simulink model "double_pend"  (R2021a)
settings: Solver=FixedStepAuto  StartTime=0.0  StopTime=10  FixedStep=.01  RelTol=1e-3
values from neighbouring files (symbols this model uses):
  alpha = params.test_25(7,1).Value    [no_exo.m]    (also in non_same_length.m = [15,15]; play_file.m = params.test_22(7,1).Value; play_file22.m = params.test_22(7,1).Value; play_file23.m = params.test_23(7,1).Value)
  beta = params.test_25(5,1).Value    [no_exo.m]    (also in non_same_length.m = [ 1/8 ; 1/8]; play_file.m = params.test_22(5,1).Value; play_file22.m = params.test_22(5,1).Value; play_file23.m = params.test_23(5,1).Value)
  Bn0 = params.test_25(1,1).Value    [no_exo.m]    (also in non_same_length.m = [500  500]; play_file.m = params.test_22(1,1).Value; play_file22.m = params.test_22(1,1).Value; play_file23.m = params.test_23(1,1).Value)
  Bp0 = params.test_25(2,1).Value    [no_exo.m]    (also in non_same_length.m = [500  500]; play_file.m = params.test_22(2,1).Value; play_file22.m = params.test_22(2,1).Value; play_file23.m = params.test_23(2,1).Value)
  dampener = [100, 0; 0, 100]    [no_exo.m]    (also in non_same_length.m; play_file.m; play_file22.m; play_file23.m)
  Dm1 = [1000,0;0,103.228187679703]    [no_exo.m]    (also in non_same_length.m = [30,0;0,30]; play_file.m = [30,0;0,30]; play_file22.m = [300,0;0,300]; play_file23.m = [30,0;0,30])
  exo_sat = 0.0    (= 0)    [no_exo.m]    (also in non_same_length.m = 150; play_file.m = 150; play_file22.m = 150; play_file23.m = 150)
  gamma = params.test_25(9,1).Value    [no_exo.m]    (also in non_same_length.m = [15,15]; play_file.m = params.test_22(9,1).Value; play_file22.m = params.test_22(9,1).Value; play_file23.m = params.test_23(9,1).Value)
  human_sat = 150    [no_exo.m]    (also in non_same_length.m = 30; play_file.m = 30; play_file22.m = 30; play_file23.m = 200)
  Ked = [ 50, 0; 0, 50]    [no_exo.m]    (also in non_same_length.m; play_file.m; play_file22.m; play_file23.m)
  Kem = [ 50, 0; 0, 50]    [no_exo.m]    (also in non_same_length.m; play_file.m; play_file22.m; play_file23.m)
  Km1 = [1000,0;0,1000]    [no_exo.m]    (also in non_same_length.m = [30, 0; 0 30]; play_file.m = [30, 0; 0 30]; play_file22.m = [300, 0; 0 300]; play_file23.m = [30, 0; 0 30])
  Kn0 = params.test_25(3,1).Value    [no_exo.m]    (also in non_same_length.m = [500  500]; play_file.m = params.test_22(3,1).Value; play_file22.m = params.test_22(3,1).Value; play_file23.m = params.test_23(3,1).Value)
  Kp0 = params.test_25(4,1).Value    [no_exo.m]    (also in non_same_length.m = [500 500]; play_file.m = params.test_22(4,1).Value; play_file22.m = params.test_22(4,1).Value; play_file23.m = params.test_23(4,1).Value)
  l = [0.324, 0.3900]    [myStateTransitionFcn.m]
  lambda2 = params.test_25(6,1).Value    [no_exo.m]    (also in non_same_length.m = [1.2, 0; 0 1.25]; play_file.m = params.test_22(6,1).Value; play_file22.m = params.test_22(6,1).Value; play_file23.m = params.test_23(6,1).Value)
  le = [0.324, 0.3900]    [no_exo.m]    (also in non_same_length.m; play_file.m; play_file22.m; play_file23.m)
  lh = [0.324, 0.3900]    [no_exo.m]    (also in non_same_length.m; play_file.m; play_file22.m; play_file23.m)
  Md = [10.0, 0; 0, 10.0]    [no_exo.m]    (also in non_same_length.m; play_file.m; play_file22.m; play_file23.m)
  me = [ 2.11, 1.28]  + mh    [no_exo.m]    (also in non_same_length.m; play_file.m; play_file22.m; play_file23.m)
  mh = [11.824, 3.848]    [no_exo.m]    (also in non_same_length.m; play_file.m; play_file22.m; play_file23.m)
  rho2 = params.test_25(8,1).Value    [no_exo.m]    (also in non_same_length.m = [100, 0; 0, 450]; play_file.m = params.test_22(8,1).Value; play_file22.m = params.test_22(8,1).Value; play_file23.m = params.test_23(8,1).Value)
  spring = [100, 0; 0, 100]    [no_exo.m]    (also in non_same_length.m; play_file.m; play_file22.m; play_file23.m)
undefined symbols (not defined in the file or in its folder): l1, l2, me2
libraries: sharedTrackingLibrary x2, simulink x2, robotcorelib x1
settings Model: Creator=nathanielgoldfarb  LastModifiedBy=nathanielgoldfarb
settings SolverCC: AlgebraicLoopSolver=TrustRegion
settings DataIOCC: ReturnWorkspaceOutputsName=SDOSimTest_Log
settings DebuggingCC: SFMachineParentedDataDiag=warning

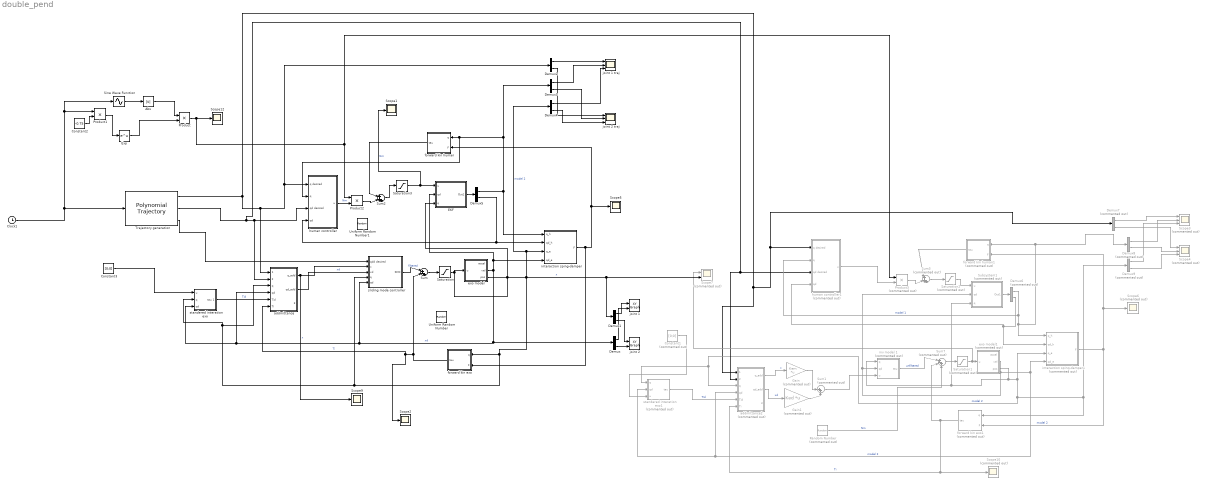
== system double_pend ==
  " interaction sping-damper" : Subsystem
  " interaction sping-damper1" : Subsystem  Commented=on
  Abs : Abs
  Clock1 : Clock
  Constant1 : Constant  Commented=on  Value=[0;0]
  Constant2 : Constant  Value=-0.75
  Constant3 : Constant  Value=[0;0]
  Demux{,1..5} (6 alike) : Demux  Outputs=2
  Demux{6..9} (4 alike) : Demux  Commented=on  Outputs=2
  EKF : Subsystem
  Exp : Math  SaturateOnIntegerOverflow=on
  Gain : Gain  Commented=on  Gain=Kem  Multiplication=Matrix(K*u)
  Gain1 : Gain  Commented=on  Gain=Ked  Multiplication=Matrix(K*u)
  Product : Product
  Product1 : Product
  Product2 : Product
  Product3 : Product  Commented=on
  Random Number : RandomNumber  Commented=on  Variance=15  SampleTime=0.1
  Saturation : Saturate  UpperLimit=exo_sat  LowerLimit=-exo_sat
  Saturation1 : Saturate  Commented=on  UpperLimit=exo_sat  LowerLimit=-exo_sat
  Saturation2 : Saturate  Commented=on  UpperLimit=human_sat  LowerLimit=-human_sat
  Saturation3 : Saturate  UpperLimit=human_sat  LowerLimit=-human_sat
  Scope{1..2,5,9,12} (5 alike) : Scope
  Scope10 : Scope  Commented=on
  Scope3 : Scope  Commented=on  NumInputPorts=3
  Scope4 : Scope  Commented=on  NumInputPorts=3
  Scope6 : Scope  Commented=on
  Scope7 : Scope  Commented=on  NumInputPorts=2
  Sine Wave Function : Sin  TimeSource=Use external signal  Frequency=5  SampleTime=0
  Subsystem1 : Subsystem  Commented=on
  Sum : Sum  Inputs=|+-+
  Sum1 : Sum  Commented=on  Inputs=|++
  Sum2 : Sum  Inputs=|+++
  Sum3 : Sum  Commented=on  Inputs=|+++
  Sum7 : Sum  Commented=on  Inputs=|+-+
  Trajectory generation : robotcorelib/Polynomial Trajectory  WaypointSource=Internal  Waypoints="[ 0 , -pi, 0;  0 -0.5*pi,0 ]"  TimePoints=[ 0, 5, 10]  TimeInterval=[ 1, 4 ]  Method=Cubic Polynomial  ParameterSource=Internal  VelocityBoundaryCondition=zeros( 2, 3 )  AccelerationBoundaryCondition=zeros( 2, 5 )  SimulateUsing=Interpreted execution
  Uniform Random Number : UniformRandomNumber  Minimum=-5  Maximum=5  SampleTime=0.1
  Uniform Random Number1 : UniformRandomNumber  Minimum=-5  Maximum=5  SampleTime=0.1
  addmittance : Subsystem
  addmittance2 : Subsystem  Commented=on
  exo model : Subsystem
  exo model1 : Subsystem  Commented=on
  forward kin exo : Subsystem
  forward kin exo1 : Subsystem  Commented=on
  forward kin human : Subsystem
  forward kin human1 : Subsystem  Commented=on
  human controller : Subsystem
  human controller1 : Subsystem  Commented=on
  inv model 1 : Subsystem  Commented=on
  joint 1 : simulink/Sinks/XY Graph  xmin=-15  xmax=15  ymin=-10  ymax=10  st=-1
  joint 1 traj : Scope  NumInputPorts=3
  joint 2 : simulink/Sinks/XY Graph  xmin=-10  xmax=10  ymin=-10  ymax=10  st=-1
  joint 2 traj : Scope  NumInputPorts=3
  sliding mode controller : Subsystem
  standered interation exo : Subsystem
  standered interation exo1 : Subsystem  Commented=on
  wires:
  forward kin human/1(tau) -> Sum2/1
  Demux4/2 -> joint 2 traj/3
  addmittance/2(qd_add) -> sliding mode controller/3(xd)  "xd"
  Constant1/1 -> standered interation exo1/3("u ")
  Demux9/2 -> Scope4/3
  Trajectory generation/3 -> sliding mode controller/1(qdd desired)
  addmittance2/1(q_add) -> Gain/1  "x"
  inv model 1/1("tau ") -> Sum7/1  "unfiltered"
  Demux3/1 -> joint 1 traj/2
  Clock1/1 -> Trajectory generation/1, Sine Wave Function/1, Product1/1
  Demux7/2 -> Scope4/1
  " interaction sping-damper"/1(F) -> forward kin exo/2(F), forward kin human/2(F), Scope5/1
  Demux2/1 -> joint 1 traj/1
  Gain/1 -> Sum1/1
  " interaction sping-damper1"/1(F) -> forward kin exo1/2(F), forward kin human1/2(F), Scope6/1  "model 2"
  exo model1/2(vel) -> inv model 1/2(qd), Subsystem1/2(qd), " interaction sping-damper1"/4("qd_e "), addmittance2/4(qd), standered interation exo1/2(qd)  "model 2"
  Gain1/1 -> Sum1/2
  Sum1/1 -> inv model 1/3("u ")
  Demux9/1 -> Scope3/3
  forward kin human1/1(tau) -> Sum3/1
  Sum7/1 -> Saturation1/1
  Demux4/1 -> joint 1 traj/3
  standered interation exo/1(tau 1) -> addmittance/5(Tid)  "Tid"
  Demux8/1 -> Scope3/2
  addmittance2/2(qd_add) -> Gain1/1  "xd"
  Random Number/1 -> Sum7/3  "Nm"
  Trajectory generation/1 -> addmittance/1(q desird), human controller/1(q desired), Demux2/1, addmittance2/1(q desird), human controller1/1(q desired), Demux7/1
  sliding mode controller/1(SMC) -> Sum/1  "filtered"
  exo model1/3(pos) -> Subsystem1/3(q), inv model 1/1(q), " interaction sping-damper1"/3(q_e), addmittance2/3(q), standered interation exo1/1(q), Demux9/1, forward kin exo1/1(q)  "model 2"
  Demux3/2 -> joint 2 traj/2
  Demux7/1 -> Scope3/1
  Demux6/2 -> human controller1/4(qd), " interaction sping-damper1"/2(qd_h)
  standered interation exo1/1("tau ") -> addmittance2/5(Tid)  "Tid"
  forward kin exo/1(tau) -> addmittance/6(Ti), Scope2/1, Sum/2  "Ti"
  Sum3/1 -> Saturation2/1
  Trajectory generation/2 -> addmittance2/2(qd desird), human controller1/3(qd desired), human controller/3(qd desired), addmittance/2(qd desird)
  addmittance/1(q_add) -> Scope9/1, sliding mode controller/2(x)  "x"
  Demux8/2 -> Scope4/2
  Demux6/1 -> " interaction sping-damper1"/1(q_h), forward kin human1/1(q), Demux8/1, human controller1/2(q)  "model 1"
  exo model/3(pos) -> Demux4/1, " interaction sping-damper"/3(q_e), sliding mode controller/4(q), standered interation exo/2(q), addmittance/3(q), forward kin exo/1(q), EKF/3(q)  "model 2"
  Demux2/2 -> joint 2 traj/1
  Demux5/1 -> Demux3/1, human controller/2(q), forward kin human/1(q), " interaction sping-damper"/1(q_h)
  Demux5/2 -> human controller/4(qd), " interaction sping-damper"/2(qd_h)
  Sum2/1 -> Saturation3/1
  EKF/1(Out1) -> Demux5/1
  Subsystem1/1(Out1) -> Demux6/1
  Sum/1 -> Saturation/1
  Saturation1/1 -> Scope7/1, exo model1/1(u)
  Saturation2/1 -> Subsystem1/1(u)
  Saturation3/1 -> Scope1/1, EKF/1(u)  "Nm"
  Abs/1 -> Product/1
  Sine Wave Function/1 -> Abs/1
  Product1/1 -> Exp/1
  Constant2/1 -> Product1/2
  Exp/1 -> Product/2
  human controller/1(u) -> Product2/2  "Nm"
  Product2/1 -> Sum2/2
  human controller1/1(u) -> Product3/2
  Product3/1 -> Sum3/2
  Product/1 -> Product2/1, Product3/1, Scope12/1
  forward kin exo1/1(tau) -> Sum7/2, addmittance2/6(Ti), Scope10/1  "Ti"
  Constant3/1 -> standered interation exo/1(u)
  Demux/2 -> joint 2/2
  Saturation/1 -> Demux1/1, Scope7/2, exo model/1(u)  "x"
  Demux1/2 -> joint 2/1
  Demux1/1 -> joint 1/1
  exo model/2(vel) -> Demux/1, addmittance/4(qd), standered interation exo/3(qd), sliding mode controller/5(qd), EKF/2(qd), " interaction sping-damper"/4("qd_e ")  "xd"
  Demux/1 -> joint 1/2

== system double_pend/ interaction sping-damper ==
  q_h : Inport
  qd_h : Inport  Port=2
  q_e : Inport  Port=3
  "qd_e " : Inport  Port=4
  Mux : Mux  Inputs=2
  Subsystem : Subsystem
  Subsystem1 : Subsystem
  forward kin : Subsystem
  forward kin1 : Subsystem
  F : Outport
  wires:
  qd_h/1 -> forward kin/2(qd)
  q_h/1 -> forward kin/1("q ")
  "qd_e "/1 -> forward kin1/2(qd)
  q_e/1 -> forward kin1/1("q ")
  forward kin/1(pos1) -> Subsystem/1(x human)
  forward kin/3(vel1) -> Subsystem/2("xd human ")
  forward kin1/1(pos1) -> Subsystem/3(x exo)
  forward kin1/3(vel1) -> Subsystem/4(xd exo)
  forward kin/2(pos2) -> Subsystem1/1(x human)
  forward kin1/2(pos2) -> Subsystem1/3(x exo)
  forward kin/4(vel2) -> Subsystem1/2("xd human ")
  forward kin1/4(vel2) -> Subsystem1/4(xd exo)
  Subsystem/1(F) -> Mux/1
  Subsystem1/1(F) -> Mux/2
  Mux/1 -> F/1

== system double_pend/ interaction sping-damper1 ==
  q_h : Inport
  qd_h : Inport  Port=2
  q_e : Inport  Port=3
  "qd_e " : Inport  Port=4
  Mux : Mux  Inputs=2
  Subsystem : Subsystem
  Subsystem1 : Subsystem
  forward kin : Subsystem
  forward kin2 : Subsystem
  F : Outport
  wires:
  qd_h/1 -> forward kin/2(qd)
  q_h/1 -> forward kin/1("q ")
  "qd_e "/1 -> forward kin2/2(qd)
  q_e/1 -> forward kin2/1("q ")
  forward kin/1(pos1) -> Subsystem/1(x human)
  forward kin/3(vel1) -> Subsystem/2("xd human ")
  forward kin2/1(pos1) -> Subsystem/3(x exo)
  forward kin2/3(vel1) -> Subsystem/4(xd exo)
  forward kin/2(pos2) -> Subsystem1/1(x human)
  forward kin2/2(pos2) -> Subsystem1/3(x exo)
  forward kin/4(vel2) -> Subsystem1/2("xd human ")
  forward kin2/4(vel2) -> Subsystem1/4(xd exo)
  Subsystem/1(F) -> Mux/1
  Subsystem1/1(F) -> Mux/2
  Mux/1 -> F/1

== system double_pend/EKF ==
  u : Inport
  qd : Inport  Port=2
  q : Inport  Port=3
  Constant5 : Constant
  Extended Kalman Filter : sharedTrackingLibrary/Extended Kalman Filter  StateTransitionFcn=myStateTransitionFcn  HasStateTransitionJacobianFcn=off  HasAdditiveProcessNoise=Additive  ProcessNoise=myQ  HasTimeVaryingProcessNoise=off  HasStateTransitionFcnExtraArgument=1  InitialState=[0;0;0;0]  InitialStateCovariance=1  MeasurementFcn1=myMeasurementFcn  HasMeasurementJacobianFcn1=off  HasMeasurementEnablePort1=on  HasAdditiveMeasurementNoise1=Additive  MeasurementNoise1=myR  HasTimeVaryingMeasurementNoise1=off  HasMeasurementFcnExtraArgument1=0  MeasurementFcn2=myMeasurementFcn  HasMeasurementJacobianFcn2=off  HasMeasurementEnablePort2=off  HasAdditiveMeasurementNoise2=Additive  MeasurementNoise2=1  HasTimeVaryingMeasurementNoise2=off  HasMeasurementFcnExtraArgument2=0  MeasurementFcn3=myMeasurementFcn  HasMeasurementJacobianFcn3=off  HasMeasurementEnablePort3=off  HasAdditiveMeasurementNoise3=Additive  MeasurementNoise3=1  HasTimeVaryingMeasurementNoise3=off  HasMeasurementFcnExtraArgument3=0  MeasurementFcn4=myMeasurementFcn  HasMeasurementJacobianFcn4=off  HasMeasurementEnablePort4=off  HasAdditiveMeasurementNoise4=Additive  MeasurementNoise4=1  HasTimeVaryingMeasurementNoise4=off  HasMeasurementFcnExtraArgument4=0  MeasurementFcn5=myMeasurementFcn  HasMeasurementJacobianFcn5=off  HasMeasurementEnablePort5=off  HasAdditiveMeasurementNoise5=Additive  MeasurementNoise5=1  HasTimeVaryingMeasurementNoise5=off  HasMeasurementFcnExtraArgument5=0  EnableMultirate=off  StateTransitionFcnSampleTime=1  MeasurementFcn1SampleTime=1  MeasurementFcn2SampleTime=1  MeasurementFcn3SampleTime=1  MeasurementFcn4SampleTime=1  MeasurementFcn5SampleTime=1  UseCurrentEstimator=on  OutputStateCovariance=off  DataType=double  SampleTime=.01  NumberOfMeasurements=1
      settings: SourceProductBaseCode=CT,DR,TF,ID,LP,NV,AR,RO,RR,UV,VE
  Mux : Mux  Inputs=2
  Zero-Order Hold : ZeroOrderHold  SampleTime=.01
  Zero-Order Hold1 : ZeroOrderHold  SampleTime=.01
  Out1 : Outport
  wires:
  Mux/1 -> Zero-Order Hold/1
  Zero-Order Hold/1 -> Extended Kalman Filter/3
  Zero-Order Hold1/1 -> Extended Kalman Filter/1
  u/1 -> Zero-Order Hold1/1
  Constant5/1 -> Extended Kalman Filter/2
  Extended Kalman Filter/1 -> Out1/1
  q/1 -> Mux/1
  qd/1 -> Mux/2

== system double_pend/Subsystem1 ==
  u : Inport
  qd : Inport  Port=2
  q : Inport  Port=3
  Constant5 : Constant
  Extended Kalman Filter : sharedTrackingLibrary/Extended Kalman Filter  StateTransitionFcn=myStateTransitionFcn  HasStateTransitionJacobianFcn=off  HasAdditiveProcessNoise=Additive  ProcessNoise=myQ  HasTimeVaryingProcessNoise=off  HasStateTransitionFcnExtraArgument=1  InitialState=[0;0;0;0]  InitialStateCovariance=1  MeasurementFcn1=myMeasurementFcn  HasMeasurementJacobianFcn1=off  HasMeasurementEnablePort1=on  HasAdditiveMeasurementNoise1=Additive  MeasurementNoise1=myR  HasTimeVaryingMeasurementNoise1=off  HasMeasurementFcnExtraArgument1=0  MeasurementFcn2=myMeasurementFcn  HasMeasurementJacobianFcn2=off  HasMeasurementEnablePort2=off  HasAdditiveMeasurementNoise2=Additive  MeasurementNoise2=1  HasTimeVaryingMeasurementNoise2=off  HasMeasurementFcnExtraArgument2=0  MeasurementFcn3=myMeasurementFcn  HasMeasurementJacobianFcn3=off  HasMeasurementEnablePort3=off  HasAdditiveMeasurementNoise3=Additive  MeasurementNoise3=1  HasTimeVaryingMeasurementNoise3=off  HasMeasurementFcnExtraArgument3=0  MeasurementFcn4=myMeasurementFcn  HasMeasurementJacobianFcn4=off  HasMeasurementEnablePort4=off  HasAdditiveMeasurementNoise4=Additive  MeasurementNoise4=1  HasTimeVaryingMeasurementNoise4=off  HasMeasurementFcnExtraArgument4=0  MeasurementFcn5=myMeasurementFcn  HasMeasurementJacobianFcn5=off  HasMeasurementEnablePort5=off  HasAdditiveMeasurementNoise5=Additive  MeasurementNoise5=1  HasTimeVaryingMeasurementNoise5=off  HasMeasurementFcnExtraArgument5=0  EnableMultirate=off  StateTransitionFcnSampleTime=1  MeasurementFcn1SampleTime=1  MeasurementFcn2SampleTime=1  MeasurementFcn3SampleTime=1  MeasurementFcn4SampleTime=1  MeasurementFcn5SampleTime=1  UseCurrentEstimator=on  OutputStateCovariance=off  DataType=double  SampleTime=.01  NumberOfMeasurements=1
      settings: SourceProductBaseCode=CT,DR,TF,ID,LP,NV,AR,RO,RR,UV,VE
  Mux : Mux  Inputs=2
  Zero-Order Hold : ZeroOrderHold  SampleTime=.01
  Zero-Order Hold1 : ZeroOrderHold  SampleTime=.01
  Out1 : Outport
  wires:
  Mux/1 -> Zero-Order Hold/1
  Zero-Order Hold/1 -> Extended Kalman Filter/3
  Zero-Order Hold1/1 -> Extended Kalman Filter/1
  u/1 -> Zero-Order Hold1/1
  Constant5/1 -> Extended Kalman Filter/2
  Extended Kalman Filter/1 -> Out1/1
  q/1 -> Mux/1
  qd/1 -> Mux/2

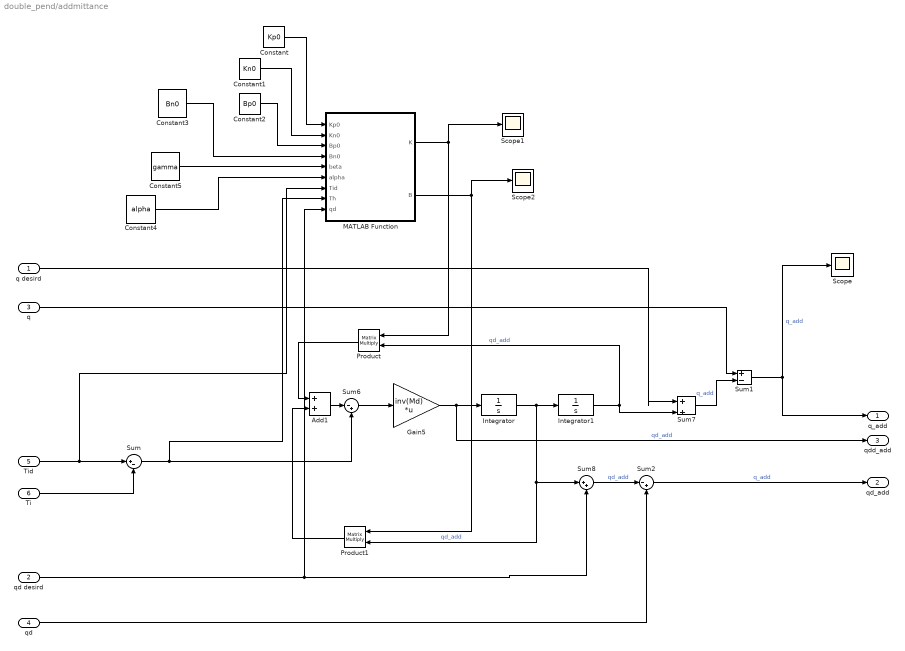
== system double_pend/addmittance ==
  q desird : Inport
  qd desird : Inport  Port=2
  q : Inport  Port=3
  qd : Inport  Port=4
  Tid : Inport  Port=5
  Ti : Inport  Port=6
  Add1 : Sum
  Constant : Constant  Value=Kp0
  Constant1 : Constant  Value=Kn0
  Constant2 : Constant  Value=Bp0
  Constant3 : Constant  Value=Bn0
  Constant4 : Constant  Value=alpha
  Constant5 : Constant  Value=gamma
  Gain5 : Gain  Gain=inv(Md)  Multiplication=Matrix(K*u)
  Integrator : Integrator
  Integrator1 : Integrator  InitialCondition=[pi;0.5*pi]
  MATLAB Function : MATLAB Function  TreatAsAtomicUnit=on
  Product : Product  Multiplication=Matrix(*)
  Product1 : Product  Multiplication=Matrix(*)
  Scope : Scope
  Scope1 : Scope
  Scope2 : Scope
  Sum : Sum  Inputs=|+-
  Sum1 : Sum  Inputs=|+-
  Sum2 : Sum  Inputs=|-+
  Sum6 : Sum  Inputs=|-+
  Sum7 : Sum  Inputs=|++
  Sum8 : Sum  Inputs=|++
  q_add : Outport
  qd_add : Outport  Port=2
  qdd_add : Outport  Port=3
  wires:
  Add1/1 -> Sum6/1
  qd desird/1 -> MATLAB Function/9(qd), Sum8/2
  Gain5/1 -> qdd_add/1, Integrator/1  "qd_add"
  Sum6/1 -> Gain5/1
  Product/1 -> Add1/1
  q desird/1 -> Sum7/1
  qd/1 -> Sum2/2
  Sum2/1 -> qd_add/1  "q_add"
  Sum7/1 -> Sum1/2  "q_add"
  q/1 -> Sum1/1
  Sum1/1 -> q_add/1, Scope/1  "q_add"
  Sum8/1 -> Sum2/1  "qd_add"
  Integrator/1 -> Product1/2, Sum8/1, Integrator1/1  "qd_add"
  Integrator1/1 -> Product/2, Sum7/2  "qd_add"
  Sum/1 -> MATLAB Function/8(Th), Sum6/2
  Tid/1 -> MATLAB Function/7(Tid), Sum/1
  Ti/1 -> Sum/2
  Product1/1 -> Add1/2
  MATLAB Function/1(K) -> Product/1, Scope1/1
  MATLAB Function/2(B) -> Product1/1, Scope2/1
  Constant/1 -> MATLAB Function/1(Kp0)
  Constant1/1 -> MATLAB Function/2(Kn0)
  Constant2/1 -> MATLAB Function/3(Bp0)
  Constant3/1 -> MATLAB Function/4(Bn0)
  Constant4/1 -> MATLAB Function/6(alpha)
  Constant5/1 -> MATLAB Function/5(beta)

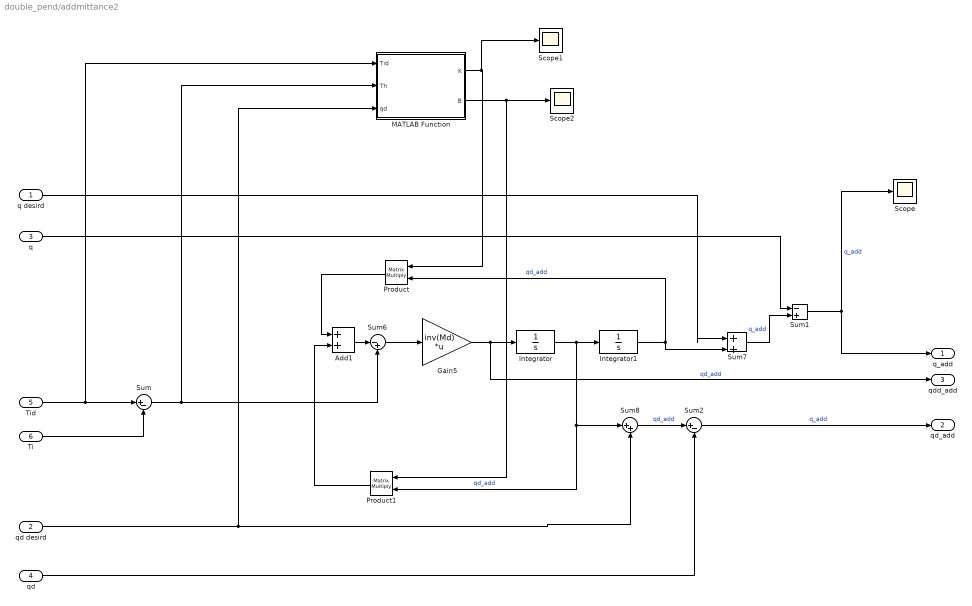
== system double_pend/addmittance2 ==
  q desird : Inport
  qd desird : Inport  Port=2
  q : Inport  Port=3
  qd : Inport  Port=4
  Tid : Inport  Port=5
  Ti : Inport  Port=6
  Add1 : Sum
  Gain5 : Gain  Gain=inv(Md)  Multiplication=Matrix(K*u)
  Integrator : Integrator
  Integrator1 : Integrator  InitialCondition=[pi;0.5*pi]
  MATLAB Function : MATLAB Function  TreatAsAtomicUnit=on
  Product : Product  Multiplication=Matrix(*)
  Product1 : Product  Multiplication=Matrix(*)
  Scope : Scope
  Scope1 : Scope
  Scope2 : Scope
  Sum : Sum  Inputs=|+-
  Sum1 : Sum  Inputs=|-+
  Sum2 : Sum  Inputs=|+-
  Sum6 : Sum  Inputs=|-+
  Sum7 : Sum  Inputs=|++
  Sum8 : Sum  Inputs=|++
  q_add : Outport
  qd_add : Outport  Port=2
  qdd_add : Outport  Port=3
  wires:
  Add1/1 -> Sum6/1
  qd desird/1 -> MATLAB Function/3(qd), Sum8/2
  Gain5/1 -> qdd_add/1, Integrator/1  "qd_add"
  Sum6/1 -> Gain5/1
  Product/1 -> Add1/1
  q desird/1 -> Sum7/1
  qd/1 -> Sum2/2
  Sum2/1 -> qd_add/1  "q_add"
  Sum7/1 -> Sum1/2  "q_add"
  q/1 -> Sum1/1
  Sum1/1 -> q_add/1, Scope/1  "q_add"
  Sum8/1 -> Sum2/1  "qd_add"
  Integrator/1 -> Product1/2, Sum8/1, Integrator1/1  "qd_add"
  Integrator1/1 -> Product/2, Sum7/2  "qd_add"
  Sum/1 -> MATLAB Function/2(Th), Sum6/2
  Tid/1 -> MATLAB Function/1(Tid), Sum/1
  Ti/1 -> Sum/2
  Product1/1 -> Add1/2
  MATLAB Function/1(K) -> Scope1/1, Product/1
  MATLAB Function/2(B) -> Scope2/1, Product1/1

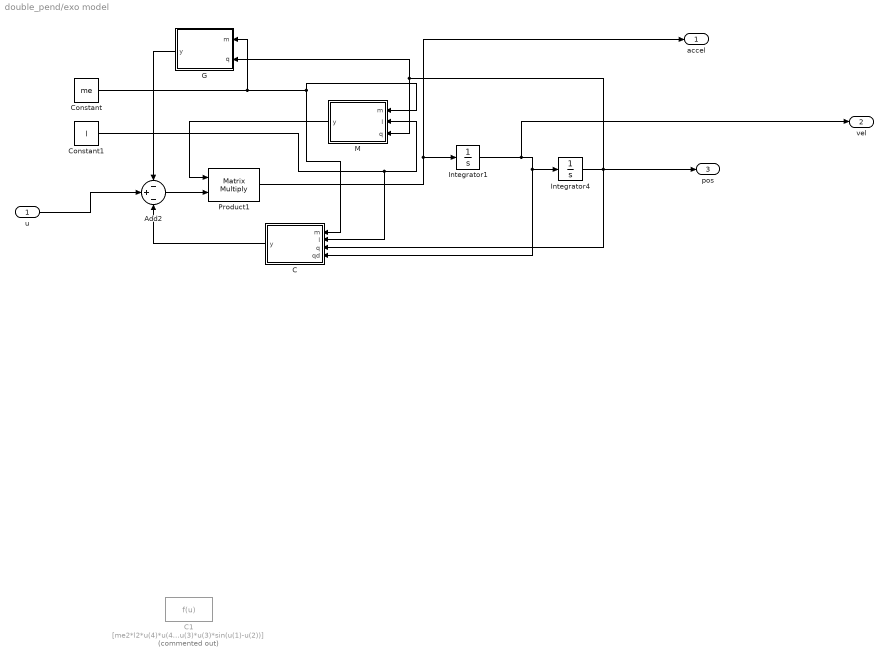
== system double_pend/exo model ==
  u : Inport
  Add2 : Sum  Inputs=-+-
  C : MATLAB Function  TreatAsAtomicUnit=on
  C1 : Fcn  Commented=on  Expr=[me2*l2*u(4)*u(4)*sin(u(1)-u(2)); -me2*l1*u(3)*u(3)*sin(u(1)-u(2))]
  Constant : Constant  Value=me
  Constant1 : Constant  Value=l
  G : MATLAB Function  TreatAsAtomicUnit=on
  Integrator1 : Integrator  InitialCondition=[0;0]
  Integrator4 : Integrator  InitialCondition=[0.01;0.01]
  M : MATLAB Function  TreatAsAtomicUnit=on
  Product1 : Product  Multiplication=Matrix(*)
  accel : Outport
  vel : Outport  Port=2
  pos : Outport  Port=3
  wires:
  Constant/1 -> G/1(m), M/1(m), C/1(m)
  M/1(y) -> Product1/1
  Add2/1 -> Product1/2
  C/1(y) -> Add2/3
  G/1(y) -> Add2/1
  u/1 -> Add2/2
  Product1/1 -> accel/1, Integrator1/1
  Constant1/1 -> C/2(l), M/2(l)
  Integrator4/1 -> C/3(q), pos/1, M/3(q), G/2(q)
  Integrator1/1 -> vel/1, C/4(qd), Integrator4/1

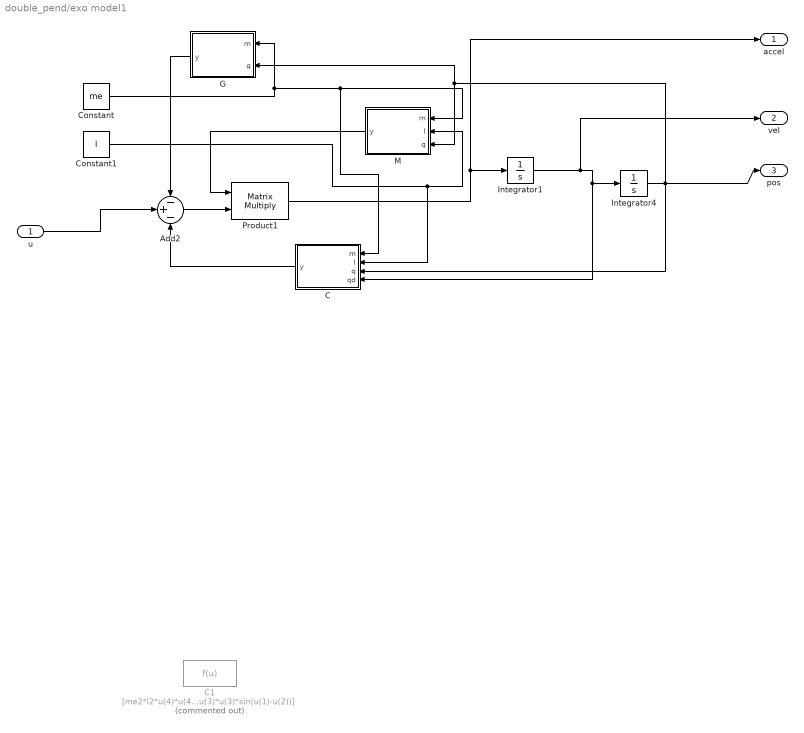
== system double_pend/exo model1 ==
  u : Inport
  Add2 : Sum  Inputs=-+-
  C : MATLAB Function  TreatAsAtomicUnit=on
  C1 : Fcn  Commented=on  Expr=[me2*l2*u(4)*u(4)*sin(u(1)-u(2)); -me2*l1*u(3)*u(3)*sin(u(1)-u(2))]
  Constant : Constant  Value=me
  Constant1 : Constant  Value=l
  G : MATLAB Function  TreatAsAtomicUnit=on
  Integrator1 : Integrator  InitialCondition=[0;0]
  Integrator4 : Integrator  InitialCondition=[0.01;0.01]
  M : MATLAB Function  TreatAsAtomicUnit=on
  Product1 : Product  Multiplication=Matrix(*)
  accel : Outport
  vel : Outport  Port=2
  pos : Outport  Port=3
  wires:
  Constant/1 -> G/1(m), C/1(m), M/1(m)
  M/1(y) -> Product1/1
  Add2/1 -> Product1/2
  C/1(y) -> Add2/3
  G/1(y) -> Add2/1
  u/1 -> Add2/2
  Product1/1 -> accel/1, Integrator1/1
  Constant1/1 -> C/2(l), M/2(l)
  Integrator1/1 -> vel/1, C/4(qd), Integrator4/1
  Integrator4/1 -> C/3(q), pos/1, M/3(q), G/2(q)

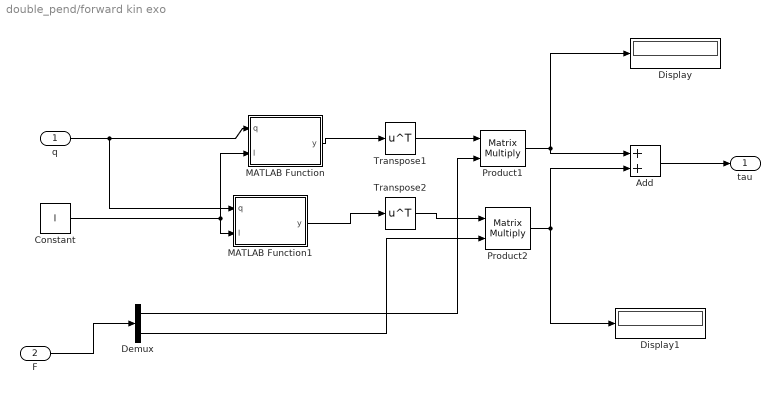
== system double_pend/forward kin exo ==
  q : Inport
  F : Inport  Port=2
  Add : Sum
  Constant : Constant  Value=l
  Demux : Demux  Outputs=2
  Display : Display
  Display1 : Display
  MATLAB Function : MATLAB Function  TreatAsAtomicUnit=on
  MATLAB Function1 : MATLAB Function  TreatAsAtomicUnit=on
  Product1 : Product  Multiplication=Matrix(*)
  Product2 : Product  Multiplication=Matrix(*)
  Transpose1 : Math  Operator=transpose  SaturateOnIntegerOverflow=on
  Transpose2 : Math  Operator=transpose  SaturateOnIntegerOverflow=on
  tau : Outport
  wires:
  Product1/1 -> Add/1, Display/1
  F/1 -> Demux/1
  q/1 -> MATLAB Function1/1(q), MATLAB Function/1(q)
  Constant/1 -> MATLAB Function/2(l), MATLAB Function1/2(l)
  Add/1 -> tau/1
  Demux/2 -> Product2/2
  Transpose2/1 -> Product2/1
  Demux/1 -> Product1/2
  Product2/1 -> Add/2, Display1/1
  MATLAB Function1/1(y) -> Transpose2/1
  MATLAB Function/1(y) -> Transpose1/1
  Transpose1/1 -> Product1/1

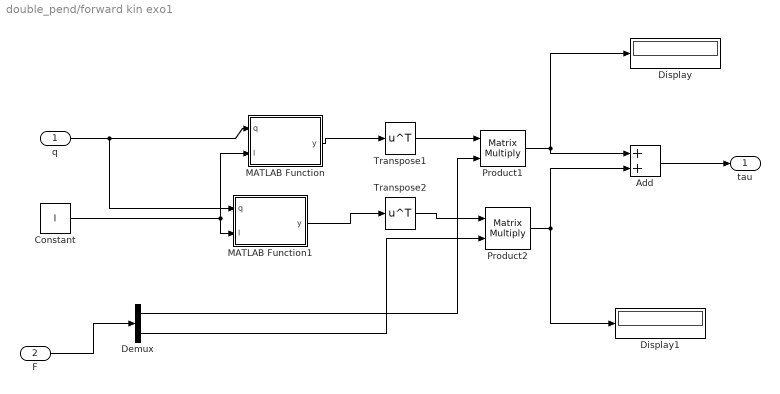
== system double_pend/forward kin exo1 ==
  q : Inport
  F : Inport  Port=2
  Add : Sum
  Constant : Constant  Value=l
  Demux : Demux  Outputs=2
  Display : Display
  Display1 : Display
  MATLAB Function : MATLAB Function  TreatAsAtomicUnit=on
  MATLAB Function1 : MATLAB Function  TreatAsAtomicUnit=on
  Product1 : Product  Multiplication=Matrix(*)
  Product2 : Product  Multiplication=Matrix(*)
  Transpose1 : Math  Operator=transpose  SaturateOnIntegerOverflow=on
  Transpose2 : Math  Operator=transpose  SaturateOnIntegerOverflow=on
  tau : Outport
  wires:
  Product1/1 -> Add/1, Display/1
  F/1 -> Demux/1
  q/1 -> MATLAB Function1/1(q), MATLAB Function/1(q)
  Constant/1 -> MATLAB Function/2(l), MATLAB Function1/2(l)
  Add/1 -> tau/1
  Demux/2 -> Product2/2
  Transpose2/1 -> Product2/1
  Demux/1 -> Product1/2
  Product2/1 -> Add/2, Display1/1
  MATLAB Function1/1(y) -> Transpose2/1
  MATLAB Function/1(y) -> Transpose1/1
  Transpose1/1 -> Product1/1

== system double_pend/forward kin human ==
  q : Inport
  F : Inport  Port=2
  Add : Sum
  Constant : Constant  Value=l
  Demux : Demux  Outputs=2
  Display : Display
  Display1 : Display
  MATLAB Function : MATLAB Function  TreatAsAtomicUnit=on
  MATLAB Function1 : MATLAB Function  TreatAsAtomicUnit=on
  Product1 : Product  Multiplication=Matrix(*)
  Product2 : Product  Multiplication=Matrix(*)
  Transpose1 : Math  Operator=transpose  SaturateOnIntegerOverflow=on
  Transpose2 : Math  Operator=transpose  SaturateOnIntegerOverflow=on
  tau : Outport
  wires:
  q/1 -> MATLAB Function1/1(q), MATLAB Function/1(q)
  Demux/2 -> Product2/2
  F/1 -> Demux/1
  Demux/1 -> Product1/2
  Transpose1/1 -> Product1/1
  Transpose2/1 -> Product2/1
  MATLAB Function1/1(y) -> Transpose2/1
  MATLAB Function/1(y) -> Transpose1/1
  Constant/1 -> MATLAB Function/2(l), MATLAB Function1/2(l)
  Add/1 -> tau/1
  Product1/1 -> Add/1, Display/1
  Product2/1 -> Add/2, Display1/1

== system double_pend/forward kin human1 ==
  q : Inport
  F : Inport  Port=2
  Add : Sum
  Constant : Constant  Value=l
  Demux : Demux  Outputs=2
  Display : Display
  Display1 : Display
  MATLAB Function : MATLAB Function  TreatAsAtomicUnit=on
  MATLAB Function1 : MATLAB Function  TreatAsAtomicUnit=on
  Product1 : Product  Multiplication=Matrix(*)
  Product2 : Product  Multiplication=Matrix(*)
  Transpose1 : Math  Operator=transpose  SaturateOnIntegerOverflow=on
  Transpose2 : Math  Operator=transpose  SaturateOnIntegerOverflow=on
  tau : Outport
  wires:
  q/1 -> MATLAB Function1/1(q), MATLAB Function/1(q)
  Demux/2 -> Product2/2
  F/1 -> Demux/1
  Demux/1 -> Product1/2
  Transpose1/1 -> Product1/1
  Transpose2/1 -> Product2/1
  MATLAB Function1/1(y) -> Transpose2/1
  MATLAB Function/1(y) -> Transpose1/1
  Constant/1 -> MATLAB Function/2(l), MATLAB Function1/2(l)
  Add/1 -> tau/1
  Product1/1 -> Add/1, Display/1
  Product2/1 -> Add/2, Display1/1

== system double_pend/human controller ==
  q desired : Inport
  q : Inport  Port=2
  qd desired : Inport  Port=3
  qd : Inport  Port=4
  Add2 : Sum
  Gain1 : Gain  Gain=Km1  Multiplication=Matrix(K*u)
  Gain2 : Gain  Gain=Dm1  Multiplication=Matrix(K*u)
  Scope2 : Scope  NumInputPorts=3
  Sum1 : Sum  Inputs=|+-
  Sum3 : Sum  Inputs=|-+
  inv model 2 : Subsystem  Commented=on
  u : Outport
  wires:
  Sum1/1 -> Gain2/1
  qd/1 -> Sum1/2
  Sum3/1 -> Gain1/1
  Gain2/1 -> Add2/2
  q desired/1 -> Sum3/2
  Gain1/1 -> Add2/1
  qd desired/1 -> Sum1/1
  q/1 -> Sum3/1
  Add2/1 -> u/1  "filtered"

== system double_pend/human controller1 ==
  q desired : Inport
  q : Inport  Port=2
  qd desired : Inport  Port=3
  qd : Inport  Port=4
  Add2 : Sum
  Gain1 : Gain  Gain=Km1  Multiplication=Matrix(K*u)
  Gain2 : Gain  Gain=Dm1  Multiplication=Matrix(K*u)
  Sum1 : Sum  Inputs=|+-
  Sum3 : Sum  Inputs=|-+
  inv model 2 : Subsystem  Commented=on
  u : Outport
  wires:
  Sum1/1 -> Gain2/1
  qd/1 -> Sum1/2
  Sum3/1 -> Gain1/1
  Gain2/1 -> Add2/2
  q desired/1 -> Sum3/2
  Gain1/1 -> Add2/1
  qd desired/1 -> Sum1/1
  q/1 -> Sum3/1
  Add2/1 -> u/1  "filtered"

== system double_pend/inv model 1 ==
  q : Inport
  qd : Inport  Port=2
  "u " : Inport  Port=3
  Add2 : Sum  Inputs=+++
  C : MATLAB Function  TreatAsAtomicUnit=on
  Constant : Constant  Value=me
  Constant1 : Constant  Value=l
  G : MATLAB Function  TreatAsAtomicUnit=on
  M : MATLAB Function  TreatAsAtomicUnit=on
  Product : Product  Multiplication=Matrix(*)
  "tau " : Outport
  wires:
  G/1(y) -> Add2/3
  C/1(y) -> Add2/2
  q/1 -> G/2(q), M/3(q), C/3(q)
  qd/1 -> C/4(qd)
  M/1(y) -> Product/1
  Product/1 -> Add2/1
  Constant/1 -> G/1(m), M/1(m), C/1(m)
  Constant1/1 -> M/2(l), C/2(l)
  "u "/1 -> Product/2
  Add2/1 -> "tau "/1

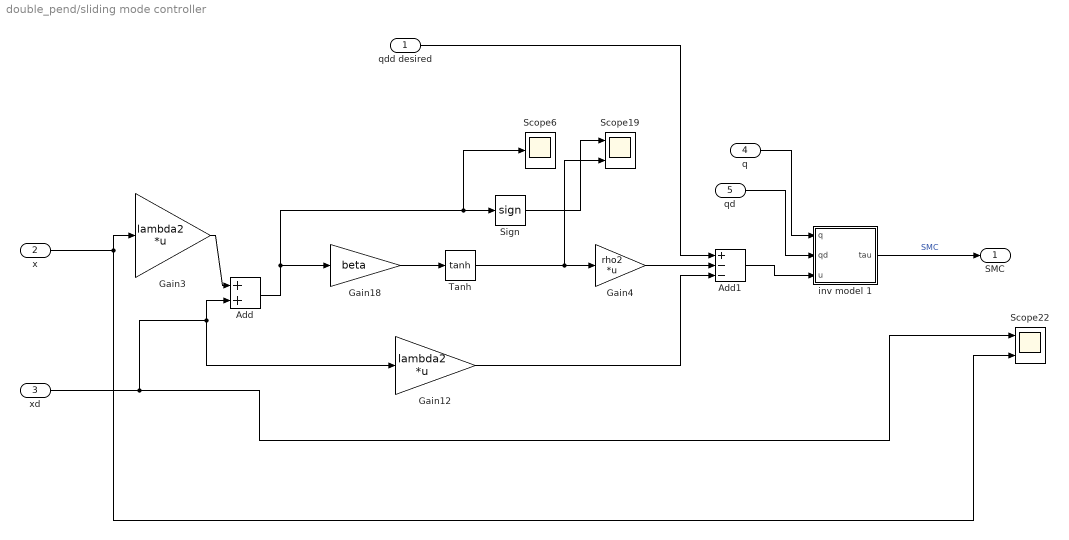
== system double_pend/sliding mode controller ==
  qdd desired : Inport
  x : Inport  Port=2
  xd : Inport  Port=3
  q : Inport  Port=4
  qd : Inport  Port=5
  Add : Sum
  Add1 : Sum  Inputs=+--
  Gain12 : Gain  Gain=lambda2  Multiplication=Matrix(K*u)
  Gain18 : Gain  Gain=beta
  Gain3 : Gain  Gain=lambda2  Multiplication=Matrix(K*u)
  Gain4 : Gain  Gain=rho2  Multiplication=Matrix(K*u)
  Scope19 : Scope  NumInputPorts=2
  Scope22 : Scope  NumInputPorts=2
  Scope6 : Scope
  Sign : Signum
  Tanh : Trigonometry  Operator=tanh
  inv model 1 : Subsystem
  SMC : Outport
  wires:
  Gain18/1 -> Tanh/1
  Gain12/1 -> Add1/3
  Gain3/1 -> Add/1
  inv model 1/1("tau ") -> SMC/1  "SMC"
  x/1 -> Scope22/2, Gain3/1
  xd/1 -> Add/2, Gain12/1, Scope22/1
  Add/1 -> Scope6/1, Sign/1, Gain18/1
  Add1/1 -> inv model 1/3("u ")
  Sign/1 -> Scope19/1
  Gain4/1 -> Add1/2
  qdd desired/1 -> Add1/1
  Tanh/1 -> Gain4/1, Scope19/2
  q/1 -> inv model 1/1(q)
  qd/1 -> inv model 1/2(qd)

== system double_pend/standered interation exo ==
  u : Inport
  q : Inport  Port=2
  qd : Inport  Port=3
  Add1 : Sum  Inputs=+++
  C : MATLAB Function  TreatAsAtomicUnit=on
  Constant2 : Constant  Value=mh
  Constant3 : Constant  Value=l
  G : MATLAB Function  TreatAsAtomicUnit=on
  M1 : MATLAB Function  TreatAsAtomicUnit=on
  Product1 : Product  Multiplication=Matrix(*)
  tau 1 : Outport
  wires:
  G/1(y) -> Add1/3
  q/1 -> G/2(q), C/3(q), M1/3(q)
  Product1/1 -> Add1/1
  Constant2/1 -> G/1(m), C/1(m), M1/1(m)
  qd/1 -> C/4(qd)
  Constant3/1 -> C/2(l), M1/2(l)
  Add1/1 -> tau 1/1
  u/1 -> Product1/2
  M1/1(y) -> Product1/1
  C/1(y) -> Add1/2

== system double_pend/standered interation exo1 ==
  q : Inport
  qd : Inport  Port=2
  "u " : Inport  Port=3
  Add2 : Sum  Inputs=+++
  C2 : MATLAB Function  TreatAsAtomicUnit=on
  Constant : Constant  Value=mh
  Constant1 : Constant  Value=l
  G1 : MATLAB Function  TreatAsAtomicUnit=on
  M : MATLAB Function  TreatAsAtomicUnit=on
  Product : Product  Multiplication=Matrix(*)
  "tau " : Outport
  wires:
  Add2/1 -> "tau "/1
  C2/1(y) -> Add2/2
  Product/1 -> Add2/1
  G1/1(y) -> Add2/3
  q/1 -> G1/2(q), C2/3(q), M/3(q)
  Constant/1 -> C2/1(m), M/1(m), G1/1(m)
  M/1(y) -> Product/1
  "u "/1 -> Product/2
  qd/1 -> C2/4(qd)
  Constant1/1 -> C2/2(l), M/2(l)

== system double_pend/ interaction sping-damper/Subsystem ==
  x human : Inport
  "xd human " : Inport  Port=2
  x exo : Inport  Port=3
  xd exo : Inport  Port=4
  Gain3 : Gain  Gain=spring  Multiplication=Matrix(K*u)
  Gain4 : Gain  Gain=dampener  Multiplication=Matrix(K*u)
  Subtract : Sum  Inputs=-+
  Subtract1 : Sum  Inputs=-+
  Subtract2 : Sum
  F : Outport
  wires:
  Subtract2/1 -> F/1
  xd exo/1 -> Subtract1/2
  Gain4/1 -> Subtract2/2
  Subtract/1 -> Gain3/1
  Subtract1/1 -> Gain4/1
  x exo/1 -> Subtract/2
  x human/1 -> Subtract/1
  "xd human "/1 -> Subtract1/1
  Gain3/1 -> Subtract2/1

== system double_pend/ interaction sping-damper/Subsystem1 ==
  x human : Inport
  "xd human " : Inport  Port=2
  x exo : Inport  Port=3
  xd exo : Inport  Port=4
  Gain3 : Gain  Gain=spring  Multiplication=Matrix(K*u)
  Gain4 : Gain  Gain=dampener  Multiplication=Matrix(K*u)
  Subtract : Sum  Inputs=-+
  Subtract1 : Sum  Inputs=-+
  Subtract2 : Sum
  F : Outport
  wires:
  Subtract2/1 -> F/1
  xd exo/1 -> Subtract1/2
  Gain4/1 -> Subtract2/2
  Subtract/1 -> Gain3/1
  Subtract1/1 -> Gain4/1
  x exo/1 -> Subtract/2
  x human/1 -> Subtract/1
  "xd human "/1 -> Subtract1/1
  Gain3/1 -> Subtract2/1

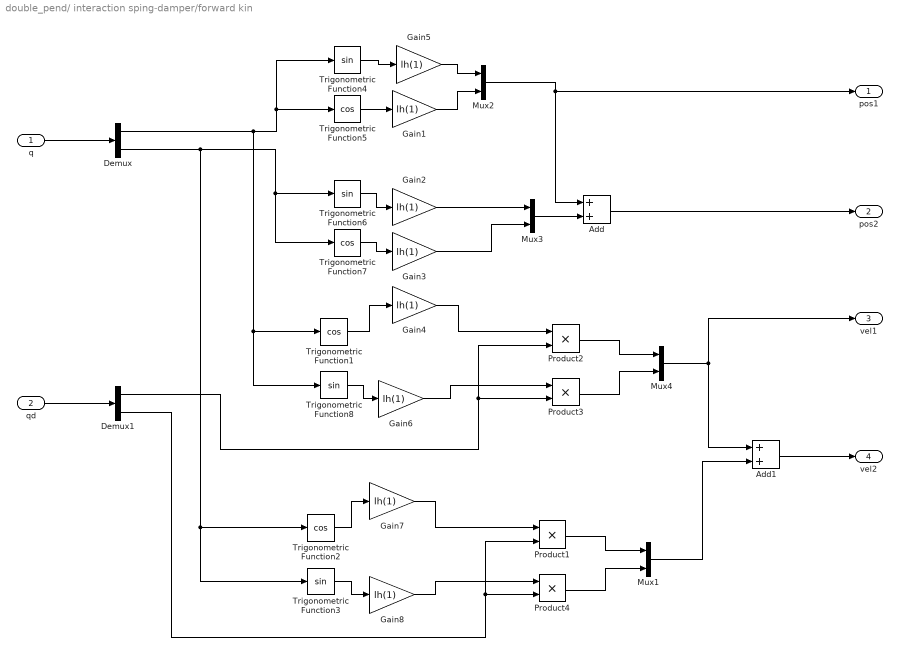
== system double_pend/ interaction sping-damper/forward kin ==
  "q " : Inport
  qd : Inport  Port=2
  Add : Sum
  Add1 : Sum
  Demux : Demux  Outputs=2
  Demux1 : Demux  Outputs=2
  Gain{1..8} (8 alike) : Gain  Gain=lh(1)
  Mux{1..4} (4 alike) : Mux  Inputs=2
  Product{1..4} (4 alike) : Product
  Trigonometric Function{1..2,5,7} (4 alike) : Trigonometry  Operator=cos
  Trigonometric Function{3..4,6,8} (4 alike) : Trigonometry
  pos1 : Outport
  pos2 : Outport  Port=2
  vel1 : Outport  Port=3
  vel2 : Outport  Port=4
  wires:
  "q "/1 -> Demux/1
  qd/1 -> Demux1/1
  Gain1/1 -> Mux2/2
  Trigonometric Function4/1 -> Gain5/1
  Gain5/1 -> Mux2/1
  Trigonometric Function5/1 -> Gain1/1
  Demux/1 -> Trigonometric Function5/1, Trigonometric Function4/1, Trigonometric Function1/1, Trigonometric Function8/1
  Trigonometric Function6/1 -> Gain2/1
  Gain3/1 -> Mux3/2
  Trigonometric Function7/1 -> Gain3/1
  Demux/2 -> Trigonometric Function3/1, Trigonometric Function2/1, Trigonometric Function7/1, Trigonometric Function6/1
  Gain2/1 -> Mux3/1
  Mux3/1 -> Add/2
  Trigonometric Function1/1 -> Gain4/1
  Gain4/1 -> Product2/1
  Demux1/1 -> Product3/2, Product2/2
  Trigonometric Function8/1 -> Gain6/1
  Gain6/1 -> Product3/1
  Product2/1 -> Mux4/1
  Product3/1 -> Mux4/2
  Trigonometric Function3/1 -> Gain8/1
  Trigonometric Function2/1 -> Gain7/1
  Product4/1 -> Mux1/2
  Demux1/2 -> Product4/2, Product1/2
  Gain8/1 -> Product4/1
  Product1/1 -> Mux1/1
  Gain7/1 -> Product1/1
  Mux4/1 -> Add1/1, vel1/1
  Mux1/1 -> Add1/2
  Add/1 -> pos2/1
  Mux2/1 -> Add/1, pos1/1
  Add1/1 -> vel2/1

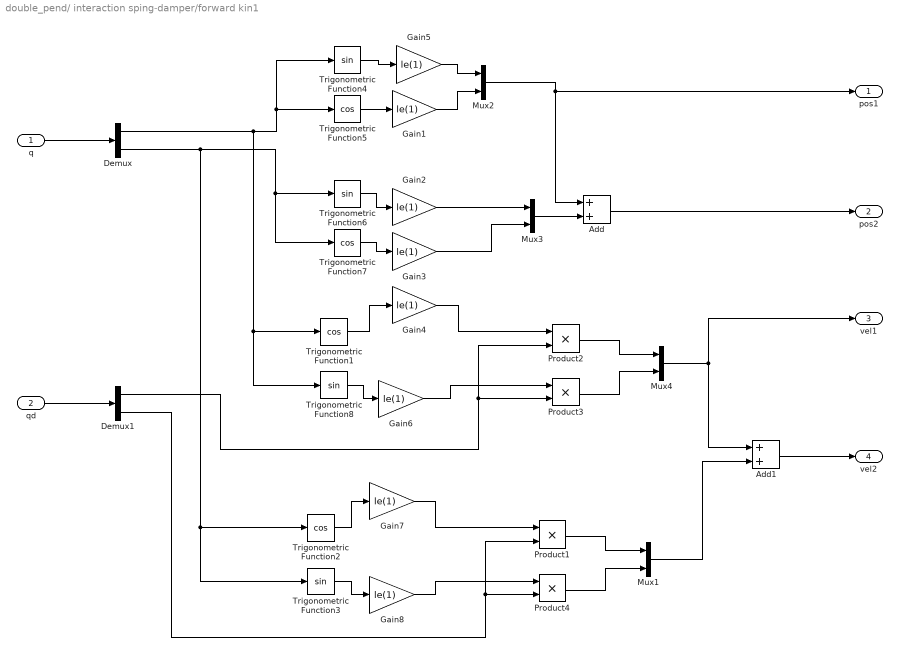
== system double_pend/ interaction sping-damper/forward kin1 ==
  "q " : Inport
  qd : Inport  Port=2
  Add : Sum
  Add1 : Sum
  Demux : Demux  Outputs=2
  Demux1 : Demux  Outputs=2
  Gain{1..8} (8 alike) : Gain  Gain=le(1)
  Mux{1..4} (4 alike) : Mux  Inputs=2
  Product{1..4} (4 alike) : Product
  Trigonometric Function{1..2,5,7} (4 alike) : Trigonometry  Operator=cos
  Trigonometric Function{3..4,6,8} (4 alike) : Trigonometry
  pos1 : Outport
  pos2 : Outport  Port=2
  vel1 : Outport  Port=3
  vel2 : Outport  Port=4
  wires:
  "q "/1 -> Demux/1
  qd/1 -> Demux1/1
  Gain1/1 -> Mux2/2
  Trigonometric Function4/1 -> Gain5/1
  Gain5/1 -> Mux2/1
  Trigonometric Function5/1 -> Gain1/1
  Demux/1 -> Trigonometric Function5/1, Trigonometric Function4/1, Trigonometric Function1/1, Trigonometric Function8/1
  Trigonometric Function6/1 -> Gain2/1
  Gain3/1 -> Mux3/2
  Trigonometric Function7/1 -> Gain3/1
  Demux/2 -> Trigonometric Function3/1, Trigonometric Function2/1, Trigonometric Function7/1, Trigonometric Function6/1
  Gain2/1 -> Mux3/1
  Mux3/1 -> Add/2
  Trigonometric Function1/1 -> Gain4/1
  Gain4/1 -> Product2/1
  Demux1/1 -> Product3/2, Product2/2
  Trigonometric Function8/1 -> Gain6/1
  Gain6/1 -> Product3/1
  Product2/1 -> Mux4/1
  Product3/1 -> Mux4/2
  Trigonometric Function3/1 -> Gain8/1
  Trigonometric Function2/1 -> Gain7/1
  Product4/1 -> Mux1/2
  Demux1/2 -> Product4/2, Product1/2
  Gain8/1 -> Product4/1
  Product1/1 -> Mux1/1
  Gain7/1 -> Product1/1
  Mux4/1 -> Add1/1, vel1/1
  Mux1/1 -> Add1/2
  Add/1 -> pos2/1
  Mux2/1 -> Add/1, pos1/1
  Add1/1 -> vel2/1

== system double_pend/ interaction sping-damper1/Subsystem ==
  x human : Inport
  "xd human " : Inport  Port=2
  x exo : Inport  Port=3
  xd exo : Inport  Port=4
  Gain3 : Gain  Gain=spring  Multiplication=Matrix(K*u)
  Gain4 : Gain  Gain=dampener  Multiplication=Matrix(K*u)
  Subtract : Sum  Inputs=-+
  Subtract1 : Sum  Inputs=-+
  Subtract2 : Sum
  F : Outport
  wires:
  Subtract2/1 -> F/1
  xd exo/1 -> Subtract1/2
  Gain4/1 -> Subtract2/2
  Subtract/1 -> Gain3/1
  Subtract1/1 -> Gain4/1
  x exo/1 -> Subtract/2
  x human/1 -> Subtract/1
  "xd human "/1 -> Subtract1/1
  Gain3/1 -> Subtract2/1

== system double_pend/ interaction sping-damper1/Subsystem1 ==
  x human : Inport
  "xd human " : Inport  Port=2
  x exo : Inport  Port=3
  xd exo : Inport  Port=4
  Gain3 : Gain  Gain=spring  Multiplication=Matrix(K*u)
  Gain4 : Gain  Gain=dampener  Multiplication=Matrix(K*u)
  Subtract : Sum  Inputs=-+
  Subtract1 : Sum  Inputs=-+
  Subtract2 : Sum
  F : Outport
  wires:
  Subtract2/1 -> F/1
  xd exo/1 -> Subtract1/2
  Gain4/1 -> Subtract2/2
  Subtract/1 -> Gain3/1
  Subtract1/1 -> Gain4/1
  x exo/1 -> Subtract/2
  x human/1 -> Subtract/1
  "xd human "/1 -> Subtract1/1
  Gain3/1 -> Subtract2/1

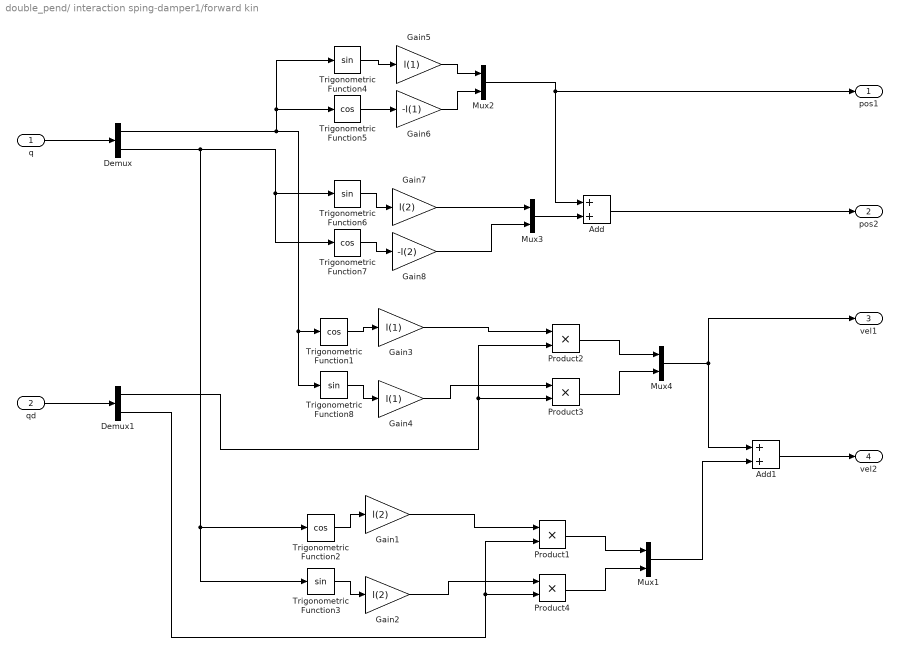
== system double_pend/ interaction sping-damper1/forward kin ==
  "q " : Inport
  qd : Inport  Port=2
  Add : Sum
  Add1 : Sum
  Demux : Demux  Outputs=2
  Demux1 : Demux  Outputs=2
  Gain1 : Gain  Gain=l(2)
  Gain2 : Gain  Gain=l(2)
  Gain3 : Gain  Gain=l(1)
  Gain4 : Gain  Gain=l(1)
  Gain5 : Gain  Gain=l(1)
  Gain6 : Gain  Gain=-l(1)
  Gain7 : Gain  Gain=l(2)
  Gain8 : Gain  Gain=-l(2)
  Mux{1..4} (4 alike) : Mux  Inputs=2
  Product{1..4} (4 alike) : Product
  Trigonometric Function{1..2,5,7} (4 alike) : Trigonometry  Operator=cos
  Trigonometric Function{3..4,6,8} (4 alike) : Trigonometry
  pos1 : Outport
  pos2 : Outport  Port=2
  vel1 : Outport  Port=3
  vel2 : Outport  Port=4
  wires:
  "q "/1 -> Demux/1
  qd/1 -> Demux1/1
  Gain6/1 -> Mux2/2
  Trigonometric Function4/1 -> Gain5/1
  Gain5/1 -> Mux2/1
  Trigonometric Function5/1 -> Gain6/1
  Demux/1 -> Trigonometric Function8/1, Trigonometric Function1/1, Trigonometric Function5/1, Trigonometric Function4/1
  Trigonometric Function6/1 -> Gain7/1
  Gain8/1 -> Mux3/2
  Trigonometric Function7/1 -> Gain8/1
  Demux/2 -> Trigonometric Function3/1, Trigonometric Function2/1, Trigonometric Function7/1, Trigonometric Function6/1
  Gain7/1 -> Mux3/1
  Mux3/1 -> Add/2
  Trigonometric Function1/1 -> Gain3/1
  Gain3/1 -> Product2/1
  Demux1/1 -> Product3/2, Product2/2
  Trigonometric Function8/1 -> Gain4/1
  Gain4/1 -> Product3/1
  Product2/1 -> Mux4/1
  Product3/1 -> Mux4/2
  Trigonometric Function3/1 -> Gain2/1
  Trigonometric Function2/1 -> Gain1/1
  Product4/1 -> Mux1/2
  Demux1/2 -> Product4/2, Product1/2
  Gain2/1 -> Product4/1
  Product1/1 -> Mux1/1
  Gain1/1 -> Product1/1
  Mux4/1 -> Add1/1, vel1/1
  Mux1/1 -> Add1/2
  Add/1 -> pos2/1
  Mux2/1 -> Add/1, pos1/1
  Add1/1 -> vel2/1

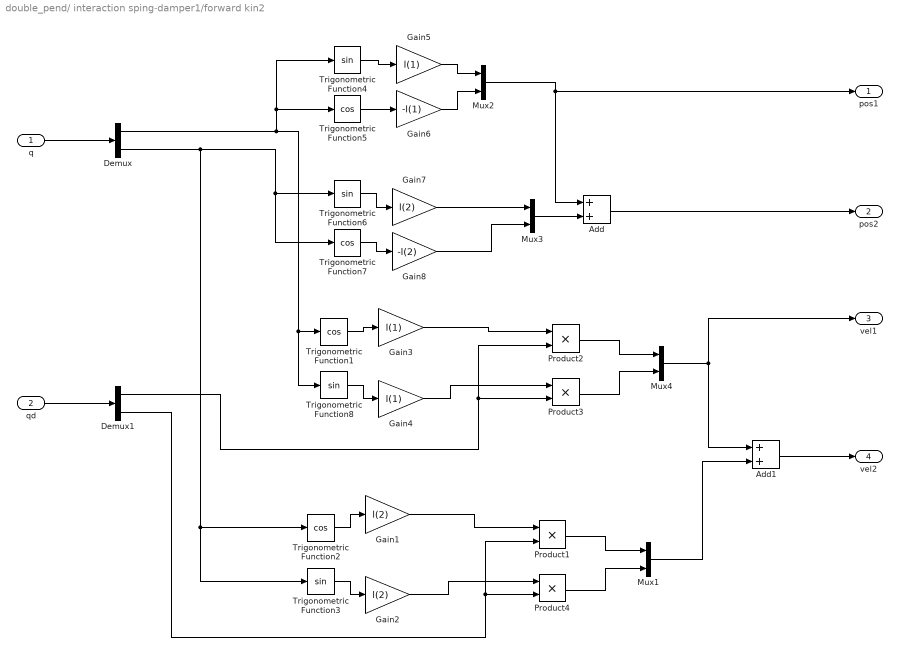
== system double_pend/ interaction sping-damper1/forward kin2 ==
  "q " : Inport
  qd : Inport  Port=2
  Add : Sum
  Add1 : Sum
  Demux : Demux  Outputs=2
  Demux1 : Demux  Outputs=2
  Gain1 : Gain  Gain=l(2)
  Gain2 : Gain  Gain=l(2)
  Gain3 : Gain  Gain=l(1)
  Gain4 : Gain  Gain=l(1)
  Gain5 : Gain  Gain=l(1)
  Gain6 : Gain  Gain=-l(1)
  Gain7 : Gain  Gain=l(2)
  Gain8 : Gain  Gain=-l(2)
  Mux{1..4} (4 alike) : Mux  Inputs=2
  Product{1..4} (4 alike) : Product
  Trigonometric Function{1..2,5,7} (4 alike) : Trigonometry  Operator=cos
  Trigonometric Function{3..4,6,8} (4 alike) : Trigonometry
  pos1 : Outport
  pos2 : Outport  Port=2
  vel1 : Outport  Port=3
  vel2 : Outport  Port=4
  wires:
  "q "/1 -> Demux/1
  qd/1 -> Demux1/1
  Gain6/1 -> Mux2/2
  Trigonometric Function4/1 -> Gain5/1
  Gain5/1 -> Mux2/1
  Trigonometric Function5/1 -> Gain6/1
  Demux/1 -> Trigonometric Function8/1, Trigonometric Function1/1, Trigonometric Function5/1, Trigonometric Function4/1
  Trigonometric Function6/1 -> Gain7/1
  Gain8/1 -> Mux3/2
  Trigonometric Function7/1 -> Gain8/1
  Demux/2 -> Trigonometric Function3/1, Trigonometric Function2/1, Trigonometric Function7/1, Trigonometric Function6/1
  Gain7/1 -> Mux3/1
  Mux3/1 -> Add/2
  Trigonometric Function1/1 -> Gain3/1
  Gain3/1 -> Product2/1
  Demux1/1 -> Product3/2, Product2/2
  Trigonometric Function8/1 -> Gain4/1
  Gain4/1 -> Product3/1
  Product2/1 -> Mux4/1
  Product3/1 -> Mux4/2
  Trigonometric Function3/1 -> Gain2/1
  Trigonometric Function2/1 -> Gain1/1
  Product4/1 -> Mux1/2
  Demux1/2 -> Product4/2, Product1/2
  Gain2/1 -> Product4/1
  Product1/1 -> Mux1/1
  Gain1/1 -> Product1/1
  Mux4/1 -> Add1/1, vel1/1
  Mux1/1 -> Add1/2
  Add/1 -> pos2/1
  Mux2/1 -> Add/1, pos1/1
  Add1/1 -> vel2/1

== system double_pend/human controller/inv model 2 ==
  q : Inport
  qd : Inport  Port=2
  "u " : Inport  Port=3
  Add2 : Sum  Inputs=+++
  C : MATLAB Function  TreatAsAtomicUnit=on
  Constant : Constant  Value=mh
  Constant1 : Constant  Value=l
  G : MATLAB Function  TreatAsAtomicUnit=on
  M : MATLAB Function  TreatAsAtomicUnit=on
  Product : Product  Multiplication=Matrix(*)
  "tau " : Outport
  wires:
  Constant1/1 -> C/2(l), M/2(l)
  Constant/1 -> G/1(m), C/1(m), M/1(m)
  "u "/1 -> Product/2
  Product/1 -> Add2/1
  M/1(y) -> Product/1
  qd/1 -> C/4(qd)
  q/1 -> G/2(q), C/3(q), M/3(q)
  Add2/1 -> "tau "/1
  C/1(y) -> Add2/2
  G/1(y) -> Add2/3

== system double_pend/human controller1/inv model 2 ==
  q : Inport
  qd : Inport  Port=2
  "u " : Inport  Port=3
  Add2 : Sum  Inputs=+++
  C : MATLAB Function  TreatAsAtomicUnit=on
  Constant : Constant  Value=mh
  Constant1 : Constant  Value=l
  G : MATLAB Function  TreatAsAtomicUnit=on
  M : MATLAB Function  TreatAsAtomicUnit=on
  Product : Product  Multiplication=Matrix(*)
  "tau " : Outport
  wires:
  Constant1/1 -> C/2(l), M/2(l)
  Constant/1 -> G/1(m), C/1(m), M/1(m)
  "u "/1 -> Product/2
  Product/1 -> Add2/1
  M/1(y) -> Product/1
  qd/1 -> C/4(qd)
  q/1 -> G/2(q), C/3(q), M/3(q)
  Add2/1 -> "tau "/1
  C/1(y) -> Add2/2
  G/1(y) -> Add2/3

== system double_pend/sliding mode controller/inv model 1 ==
  q : Inport
  qd : Inport  Port=2
  "u " : Inport  Port=3
  Add2 : Sum  Inputs=+++
  C : MATLAB Function  TreatAsAtomicUnit=on
  Constant : Constant  Value=me
  Constant1 : Constant  Value=l
  G : MATLAB Function  TreatAsAtomicUnit=on
  M : MATLAB Function  TreatAsAtomicUnit=on
  Product : Product  Multiplication=Matrix(*)
  "tau " : Outport
  wires:
  G/1(y) -> Add2/3
  C/1(y) -> Add2/2
  Add2/1 -> "tau "/1
  q/1 -> G/2(q), C/3(q), M/3(q)
  qd/1 -> C/4(qd)
  M/1(y) -> Product/1
  Product/1 -> Add2/1
  "u "/1 -> Product/2
  Constant/1 -> G/1(m), C/1(m), M/1(m)
  Constant1/1 -> C/2(l), M/2(l)

== matlab function double_pend/human controller1/inv model 2/C ==
  data: m input; l input; q input; y output; qd input
function y = fcn(m, l, q, qd)



y = C(m, l, q, qd); % [m(2)*l(2)*qd(2)*qd(2)*sin(q(1)-q(2)); -m(2)*l(1)*qd(1)*qd(1)*sin(q(1)-q(2))];

== matlab function double_pend/forward kin exo/MATLAB Function1 ==
  data: q input; y output; l input
function y = fcn(q, l)


y = [l(1)*cos(q(1)), l(2)*cos(q(2)) ; l(1)*sin(q(1)), l(2)*sin(q(2)) ];

== matlab function double_pend/forward kin human/MATLAB Function ==
  data: q input; y output; l input
function y = fcn(q,l)

y = [l(1)*cos(q(1)), 0; l(1)*sin(q(1)), 0 ];

== matlab function double_pend/forward kin human/MATLAB Function1 ==
  data: q input; y output; l input
function y = fcn(q, l)


y = [l(1)*cos(q(1)), l(2)*cos(q(2)) ; l(1)*sin(q(1)), l(2)*sin(q(2)) ];

== matlab function double_pend/exo model/C ==
  data: m input; l input; q input; y output; qd input
function y = fcn(m, l, q, qd)



y = C(m, l, q, qd); % [m(2)*l(2)*qd(2)*qd(2)*sin(q(1)-q(2)); -m(2)*l(1)*qd(1)*qd(1)*sin(q(1)-q(2))];

== matlab function double_pend/exo model/G ==
  data: m input; q input; y output
function y = fcn(m, q)
 y = [50; 50] + G(m,q);
end

== matlab function double_pend/exo model/M ==
  data: m input; l input; q input; y output
function y = fcn(m, l, q)

y = pinv(M(m,l,q)); % pinv([ (m(1)+m(2)) *l(1), m(2)*l(2)*cos(q(1)-q(2)); m(2)* l(1)*cos(q(1)-q(2)), m(2)*l(2)] );

end

== matlab function double_pend/standered interation exo/C ==
  data: m input; l input; q input; y output; qd input
function y = fcn(m, l, q, qd)



y = C(m, l, q, qd); % [m(2)*l(2)*qd(2)*qd(2)*sin(q(1)-q(2)); -m(2)*l(1)*qd(1)*qd(1)*sin(q(1)-q(2))];

== matlab function double_pend/standered interation exo/G ==
  data: m input; q input; y output
function y = fcn(m, q)
 y =  G(m,q);
end

== matlab function double_pend/standered interation exo/M1 ==
  data: m input; l input; q input; y output
function y = fcn(m, l, q)

y = M(m,l,q); % pinv([ (m(1)+m(2)) *l(1), m(2)*l(2)*cos(q(1)-q(2)); m(2)* l(1)*cos(q(1)-q(2)), m(2)*l(2)] );

end

== matlab function double_pend/human controller/inv model 2/C ==
  data: m input; l input; q input; y output; qd input
function y = fcn(m, l, q, qd)



y = C(m, l, q, qd); % [m(2)*l(2)*qd(2)*qd(2)*sin(q(1)-q(2)); -m(2)*l(1)*qd(1)*qd(1)*sin(q(1)-q(2))];

== matlab function double_pend/forward kin exo1/MATLAB Function ==
  data: q input; y output; l input
function y = fcn(q,l)

y = [l(1)*cos(q(1)), 0; l(1)*sin(q(1)), 0 ];

== matlab function double_pend/standered interation exo1/C2 ==
  data: m input; l input; q input; y output; qd input
function y = fcn(m, l, q, qd)



y = [m(2)*l(2)*qd(2)*qd(2)*sin(q(1)-q(2)); -m(2)*l(1)*qd(1)*qd(1)*sin(q(1)-q(2))];

== matlab function double_pend/standered interation exo1/G1 ==
  data: m input; q input; y output
function y = fcn(m, q)

g = 9.81;

y =[ (m(1)+m(2))*g*sin(q(1)); m(2)*g*sin(q(1))] ;

== matlab function double_pend/standered interation exo1/M ==
  data: m input; l input; q input; y output
function y = fcn(m, l, q)

y =[ (m(1)+m(2)) *l(1), m(2)*cos(q(1)-q(2)); m(2)*l(1)*cos(q(1)-q(2)), m(2)*l(2)] ;

== matlab function double_pend/human controller1/inv model 2/G ==
  data: m input; q input; y output
function y = fcn(m, q)
 y =  G(m,q);
end

== matlab function double_pend/human controller1/inv model 2/M ==
  data: m input; l input; q input; y output
function y = fcn(m, l, q)

y = M(m,l,q); % pinv([ (m(1)+m(2)) *l(1), m(2)*l(2)*cos(q(1)-q(2)); m(2)* l(1)*cos(q(1)-q(2)), m(2)*l(2)] );

end

== matlab function double_pend/forward kin exo1/MATLAB Function1 ==
  data: q input; y output; l input
function y = fcn(q, l)


y = [l(1)*cos(q(1)), l(2)*cos(q(2)) ; l(1)*sin(q(1)), l(2)*sin(q(2)) ];

== matlab function double_pend/forward kin human1/MATLAB Function ==
  data: q input; y output; l input
function y = fcn(q,l)

y = [l(1)*cos(q(1)), 0; l(1)*sin(q(1)), 0 ];

== matlab function double_pend/forward kin human1/MATLAB Function1 ==
  data: q input; y output; l input
function y = fcn(q, l)


y = [l(1)*cos(q(1)), l(2)*cos(q(2)) ; l(1)*sin(q(1)), l(2)*sin(q(2)) ];

== matlab function double_pend/inv model 1/C ==
  data: m input; l input; q input; y output; qd input
function y = fcn(m, l, q, qd)



y = C(m, l, q, qd); % [m(2)*l(2)*qd(2)*qd(2)*sin(q(1)-q(2)); -m(2)*l(1)*qd(1)*qd(1)*sin(q(1)-q(2))];

== matlab function double_pend/inv model 1/G ==
  data: m input; q input; y output
function y = fcn(m, q)
 y =  G(m,q);
end

== matlab function double_pend/inv model 1/M ==
  data: m input; l input; q input; y output
function y = fcn(m, l, q)

y = M(m,l,q); % pinv([ (m(1)+m(2)) *l(1), m(2)*l(2)*cos(q(1)-q(2)); m(2)* l(1)*cos(q(1)-q(2)), m(2)*l(2)] );

end

== matlab function double_pend/human controller/inv model 2/G ==
  data: m input; q input; y output
function y = fcn(m, q)
 y =  G(m,q);
end

== matlab function double_pend/exo model1/C ==
  data: m input; l input; q input; y output; qd input
function y = fcn(m, l, q, qd)



y = C(m, l, q, qd); % [m(2)*l(2)*qd(2)*qd(2)*sin(q(1)-q(2)); -m(2)*l(1)*qd(1)*qd(1)*sin(q(1)-q(2))];

== matlab function double_pend/exo model1/G ==
  data: m input; q input; y output
function y = fcn(m, q)
 y = [50;50] + G(m,q);
end

== matlab function double_pend/exo model1/M ==
  data: m input; l input; q input; y output
function y = fcn(m, l, q)

y = pinv( M(m,l,q)); % pinv([ (m(1)+m(2)) *l(1), m(2)*l(2)*cos(q(1)-q(2)); m(2)* l(1)*cos(q(1)-q(2)), m(2)*l(2)] );

end

== matlab function double_pend/human controller/inv model 2/M ==
  data: m input; l input; q input; y output
function y = fcn(m, l, q)

y = M(m,l,q); % pinv([ (m(1)+m(2)) *l(1), m(2)*l(2)*cos(q(1)-q(2)); m(2)* l(1)*cos(q(1)-q(2)), m(2)*l(2)] );

end

== matlab function double_pend/sliding mode controller/inv model 1/C ==
  data: m input; l input; q input; y output; qd input
function y = fcn(m, l, q, qd)



y = C(m, l, q, qd); % [m(2)*l(2)*qd(2)*qd(2)*sin(q(1)-q(2)); -m(2)*l(1)*qd(1)*qd(1)*sin(q(1)-q(2))];

== matlab function double_pend/sliding mode controller/inv model 1/G ==
  data: m input; q input; y output
function y = fcn(m, q)
 y =  G(m,q);
end

== matlab function double_pend/sliding mode controller/inv model 1/M ==
  data: m input; l input; q input; y output
function y = fcn(m, l, q)

y = M(m,l,q); % pinv([ (m(1)+m(2)) *l(1), m(2)*l(2)*cos(q(1)-q(2)); m(2)* l(1)*cos(q(1)-q(2)), m(2)*l(2)] );

end

== matlab function double_pend/forward kin exo/MATLAB Function ==
  data: q input; y output; l input
function y = fcn(q,l)

y = [l(1)*cos(q(1)), 0; l(1)*sin(q(1)), 0 ];

== matlab function double_pend/addmittance/MATLAB Function ==
  data: Kp0 input; Kn0 input; Bp0 input; Bn0 input; beta input; alpha input; Tid input; K output; Th input; qd input; B output
function [K,B] = fcn(Kp0, Kn0, Bp0, Bn0, beta, alpha,Tid, Th, qd)

Kp0 = diag(Kp0);
Kn0 = diag(Kn0);% [500 0; 0 500];
Bp0 = diag(Bp0);% [500 0; 0 500];
Bn0 =  diag(Bn0);%[500 0; 0 500];
beta_p = beta(1);
beta_n = beta(2);
alpha_p = alpha(1);
alpha_n = alpha(2);

intention = sign(Th) == sign(qd);
change = abs(Th/Tid);

K = eye(size(intention,1));
B = eye(size(intention,1));
count = 1;
my_intention = [0;0];


for ii =  1:length(intention)
   if intention(ii)
        K(count,count) = Kp0(count,count) + beta_p*change(count);
        B(count,count) = Bp0(count,count) + alpha_p*change(count);
   else
       K(count,count) = Kn0(count,count) - beta_n*change(count);
       B(count,count) = Bn0(count,count) - alpha_n*change(count);
   end
   my_intention(count) = 0;
   count= count + 1;
   

end


end

== matlab function double_pend/addmittance2/MATLAB Function ==
  data: Tid input; K output; Th input; qd input; B output
function [K,B] = fcn(Tid, Th, qd)

Kp0 = [75 0; 0 25];
Kn0 = [50 0; 0 50];
Bp0 = [75 0; 0 25];
Bn0 = [50 0; 0 50];
beta_p = 3;
beta_n = 3;
alpha_p = 0.5;
alpha_n = 0.5;

intention = sign(Th) == sign(qd);
change = abs(Th/Tid);

K = eye(size(intention,1));
B = eye(size(intention,1));
count = 1;
my_intention = [0;0];


for ii =  1:length(intention)
   if intention(ii)
        K(count,count) = Kp0(count,count) + beta_p*change(count);
        B(count,count) = Bp0(count,count) + alpha_p*change(count);
   else
       K(count,count) = Kn0(count,count) - beta_n*change(count);
       B(count,count) = Bn0(count,count) - alpha_n*change(count);
   end
   my_intention(count) = 0;
   count= count + 1;
   

end


end
